simulink model "sensor_capacitive_chain"  (R2022a)
settings: Solver=ode45  StartTime=0.0  StopTime=12  RelTol=1e-6  AbsTol=1e-8
settings Model: Creator=HJL  LastModifiedBy=HJL

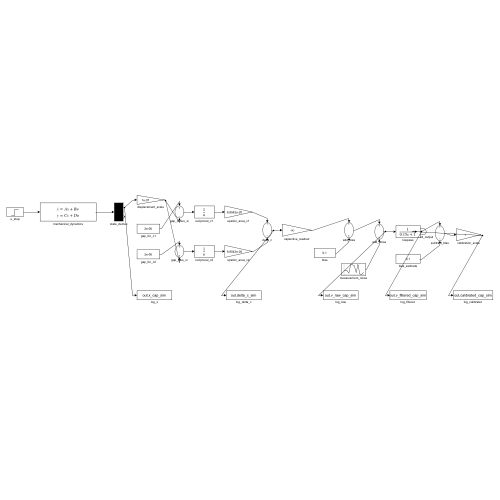
[thumbnail: Simulink's stored preview of the top-level diagram]
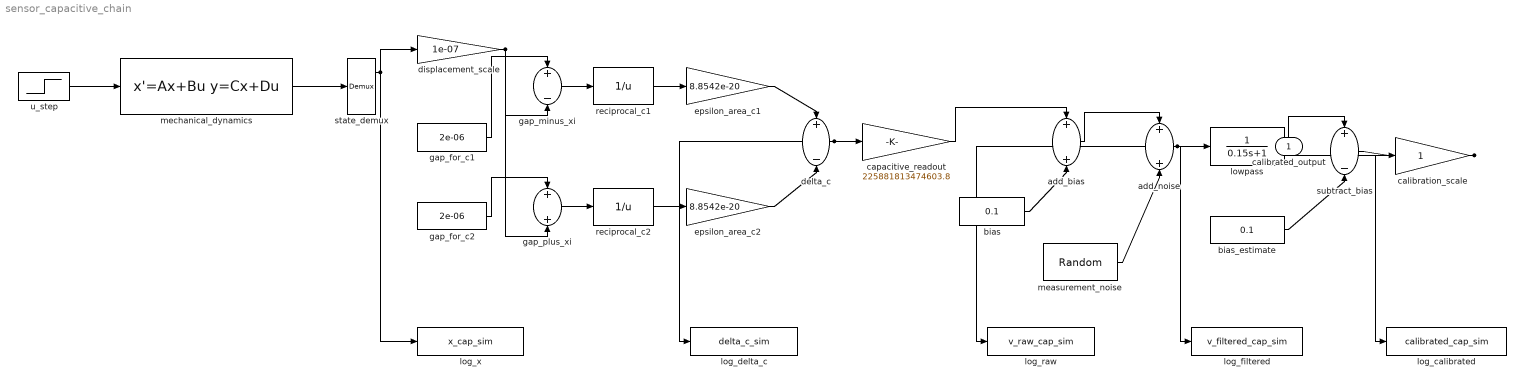
== system sensor_capacitive_chain ==
  add_bias : Sum
  add_noise : Sum
  bias : Constant  Value=0.1
  bias_estimate : Constant  Value=0.1
  calibration_scale : Gain
  capacitive_readout : Gain  Gain=225881813474603.8
  delta_c : Sum  Inputs=+-
  displacement_scale : Gain  Gain=1e-07
  epsilon_area_c1 : Gain  Gain=8.8542e-20
  epsilon_area_c2 : Gain  Gain=8.8542e-20
  gap_for_c1 : Constant  Value=2e-06
  gap_for_c2 : Constant  Value=2e-06
  gap_minus_xi : Sum  Inputs=+-
  gap_plus_xi : Sum
  log_calibrated : ToWorkspace  VariableName=calibrated_cap_sim  SaveFormat=Timeseries  SampleTime=-1
  log_delta_c : ToWorkspace  VariableName=delta_c_sim  SaveFormat=Timeseries  SampleTime=-1
  log_filtered : ToWorkspace  VariableName=v_filtered_cap_sim  SaveFormat=Timeseries  SampleTime=-1
  log_raw : ToWorkspace  VariableName=v_raw_cap_sim  SaveFormat=Timeseries  SampleTime=-1
  log_x : ToWorkspace  VariableName=x_cap_sim  SaveFormat=Timeseries  SampleTime=-1
  lowpass : TransferFcn  Denominator=[0.15 1]
  measurement_noise : RandomNumber  Variance=0.0001  Seed=7  SampleTime=0.01
  mechanical_dynamics : StateSpace  A=[0 1; -1.2 -0.2]  B=[0; 1]  C=[1 0; 0 1]  D=[0; 0]  InitialCondition=[0; 0]
  reciprocal_c1 : Math  Operator=reciprocal
  reciprocal_c2 : Math  Operator=reciprocal
  state_demux : Demux  Outputs=2
  subtract_bias : Sum  Inputs=+-
  u_step : Step  SampleTime=0
  calibrated_output : Outport
  wires:
  u_step/1 -> mechanical_dynamics/1
  mechanical_dynamics/1 -> state_demux/1
  state_demux/1 -> displacement_scale/1, log_x/1
  displacement_scale/1 -> gap_minus_xi/2, gap_plus_xi/2
  gap_for_c1/1 -> gap_minus_xi/1
  gap_for_c2/1 -> gap_plus_xi/1
  gap_minus_xi/1 -> reciprocal_c1/1
  gap_plus_xi/1 -> reciprocal_c2/1
  reciprocal_c1/1 -> epsilon_area_c1/1
  reciprocal_c2/1 -> epsilon_area_c2/1
  epsilon_area_c1/1 -> delta_c/1
  epsilon_area_c2/1 -> delta_c/2
  delta_c/1 -> capacitive_readout/1, log_delta_c/1
  capacitive_readout/1 -> add_bias/1
  bias/1 -> add_bias/2
  add_bias/1 -> add_noise/1
  measurement_noise/1 -> add_noise/2
  add_noise/1 -> lowpass/1, log_raw/1
  lowpass/1 -> subtract_bias/1, log_filtered/1
  bias_estimate/1 -> subtract_bias/2
  subtract_bias/1 -> calibration_scale/1
  calibration_scale/1 -> calibrated_output/1, log_calibrated/1
